simulink model "getting_started_paced"  (R2017b)
settings: Solver=FixedStepAuto  StartTime=0.0  StopTime=inf  FixedStep=.1  RelTol=1e-3
undefined symbols (not defined in the file): X, Y
libraries: robotlib x3, realtime_pacer_lib x1, simulink x1
settings Model: Creator=jshapiro  LastModifiedBy=jshapiro

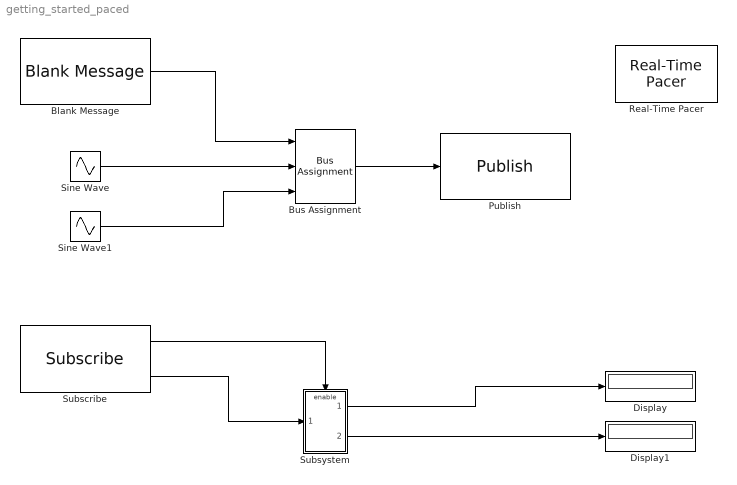
== system getting_started_paced ==
  Blank Message : robotlib/Blank Message  SourceLibraryInfo=This block requires Robotics System Toolbox  messageType=geometry_msgs/Point  SampleTime=inf
      settings: SourceProductBaseCode=RO
  Bus Assignment : BusAssignment  AssignedSignals=X,Y
  Display : Display
  Display1 : Display
  Publish : robotlib/Publish  SourceLibraryInfo=This block requires Robotics System Toolbox  topicSource=Specify your own  topic=/location  messageType=geometry_msgs/Point  messageQueueLength=1
      settings: SourceProductBaseCode=RO
  Real-Time Pacer : realtime_pacer_lib/Real-Time Pacer  simTimePerRealTime=1
  Sine Wave : Sin  Phase=-pi/2  SampleTime=0
  Sine Wave1 : Sin  SampleTime=0
  Subscribe : robotlib/Subscribe  SourceLibraryInfo=This block requires Robotics System Toolbox  topicSource=Specify your own  topic=/location  messageType=geometry_msgs/Point  sampleTime=-1  messageQueueLength=1
      settings: SourceProductBaseCode=RO
  Subsystem : Subsystem
  wires:
  Blank Message/1 -> Bus Assignment/1
  Bus Assignment/1 -> Publish/1
  Sine Wave/1 -> Bus Assignment/2
  Sine Wave1/1 -> Bus Assignment/3
  Subscribe/1 -> Subsystem/Enable
  Subscribe/2 -> Subsystem/1(In1)
  Subsystem/1(<X>) -> Display/1
  Subsystem/2(<Y>) -> Display1/1

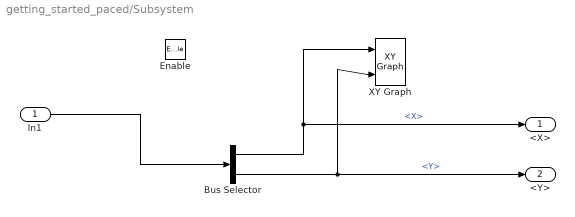
== system getting_started_paced/Subsystem ==
  In1 : Inport
  Enable : EnablePort
  Bus Selector : BusSelector  OutputSignals=X,Y
  XY Graph : simulink/Sinks/XY Graph  xmin=-1  xmax=1  ymin=-1  ymax=1  st=-1
  <X> : Outport
  <Y> : Outport  Port=2
  wires:
  Bus Selector/2 -> <Y>/1, XY Graph/2  "<Y>"
  Bus Selector/1 -> <X>/1, XY Graph/1  "<X>"
  In1/1 -> Bus Selector/1
